simulink subsystem "PieroHW"  (R2023b)
settings: Solver=VariableStepAuto  StartTime=0.0  StopTime=10.0  RelTol=1e-3
libraries: simulink x1
settings Model: Creator=Usuario_UMA  LastModifiedBy=Usuario_UMA

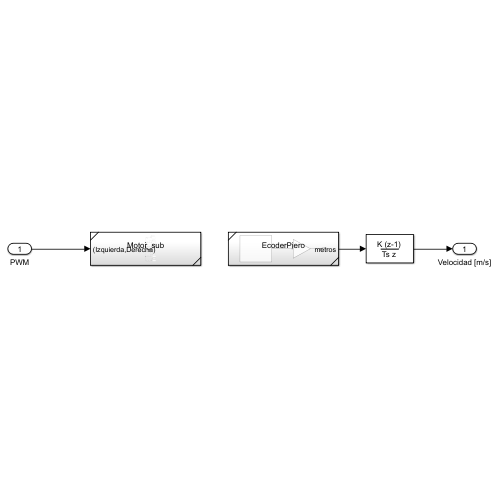
[thumbnail: Simulink's stored preview of the top-level diagram]
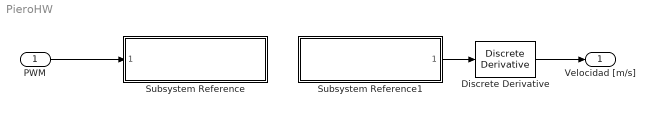
== system PieroHW ==
  PWM : Inport
  Discrete Derivative : simulink/Discrete/Discrete Derivative  gainval=1.0  ICPrevScaledInput=0.0  OutMin=[]  OutMax=[]  OutDataType=fixdt(1, 16)  OutScaling=2^-10  DoSatur=off
  Subsystem Reference : Subsystem  ReferencedSubsystem=Motor_sub
  Subsystem Reference1 : Subsystem  ReferencedSubsystem=EcoderPiero
  Velocidad [m/s] : Outport
  wires:
  PWM/1 -> Subsystem Reference/1
  Discrete Derivative/1 -> Velocidad [m/s]/1
  Subsystem Reference1/1 -> Discrete Derivative/1
